simulink model "cosim_der2"  (R2021b)
settings: Solver=VariableStepAuto  StartTime=0.0  StopTime=inf  FixedStep=1e-3  RelTol=1e-3
values from neighbouring files (symbols this model uses):
  data_in = [0.785293830964 0.808251211481 0.30791492871 0.0344445946687 0.179843791508 0.360027135025 0.556566365757 0.556566365757 0.360027135025 0.179843791508 0.0344445946687 0.30791492871 ... (14 elements, 2x7)]    [caca.mat]    (also in cosim1.m = readmatrix("data_in1.csv"); cosim2.m = readmatrix("data_in2.csv"))
undefined symbols (not defined in the file or in its folder): xc7vx485tffg1157
libraries: hdlBasic x14, hdlSSR x1, vmcUtilities x1
settings Model: Creator=fabus  LastModifiedBy=fabus
settings DataIOCC: ExternalInput=data_in

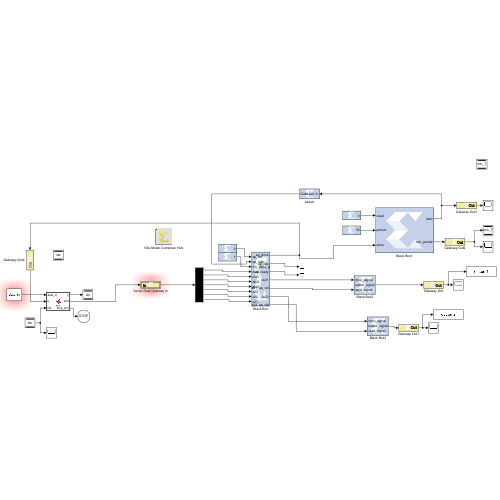
[thumbnail: Simulink's stored preview of the top-level diagram]
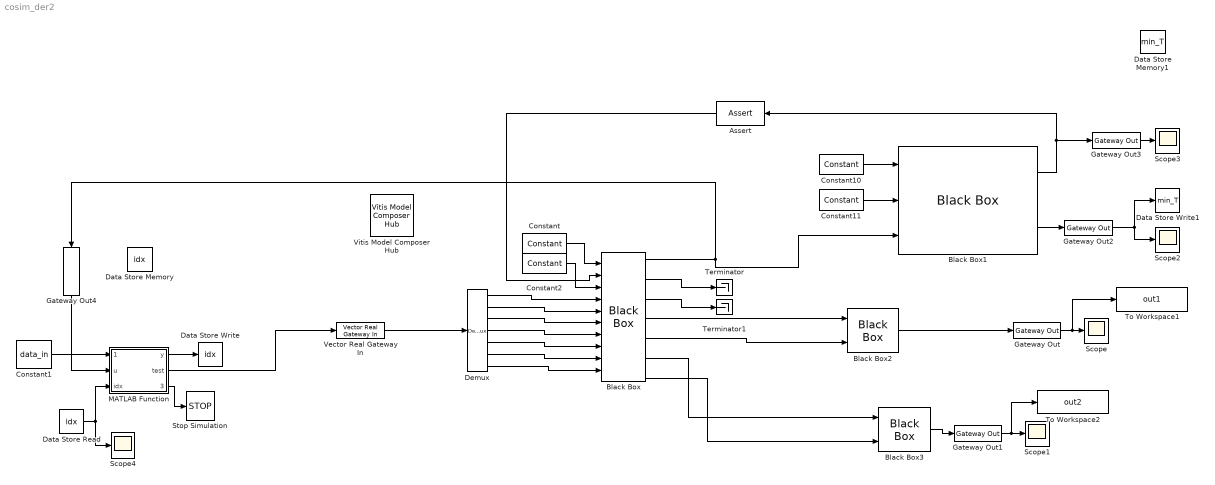
== system cosim_der2 ==
  Assert : hdlBasic/Assert  assert_type=off  type_source=Explicitly  gui_display_data_type=Fixed-point  arith_type=Signed (2's comp)  n_bits=16  bin_pt=14  preci_type=Single  exp_width=8  frac_width=24  assert_rate=on  rate_source=Explicitly  period=1  output_port=on  XmcBlockStatus=1  maskContainerNames=group1  block_type=assert  block_config=sysgen:assert_config  block_width=609  block_height=900
  Black Box : hdlBasic/Black Box  init_code=der2_config  sim_method=Vivado Simulator  verbose=off  XmcBlockStatus=1  maskContainerNames=group1  block_type=blackbox2  block_config=sysgen:black_box_config
  Black Box1 : hdlBasic/Black Box  init_code=period_setter_config  sim_method=Vivado Simulator  verbose=off  XmcBlockStatus=1  maskContainerNames=group1  block_type=blackbox2  block_config=sysgen:black_box_config
  Black Box2 : hdlBasic/Black Box  init_code=valid_out15_config  sim_method=Vivado Simulator  verbose=off  XmcBlockStatus=1  maskContainerNames=group1  block_type=blackbox2  block_config=sysgen:black_box_config
  Black Box3 : hdlBasic/Black Box  init_code=valid_out15_config  sim_method=Vivado Simulator  verbose=off  XmcBlockStatus=1  maskContainerNames=group1  block_type=blackbox2  block_config=sysgen:black_box_config
  Constant : hdlBasic/Constant  const=0  gui_display_data_type=Fixed-point  arith_type=Unsigned  n_bits=1  bin_pt=0  preci_type=Single  exp_width=8  frac_width=24  explicit_period=off  period=1  XmcBlockStatus=1  maskContainerNames=tabcontainer1  block_type=constant  block_config=sysgen:Constant_config
  Constant1 : Constant  Value=data_in
  Constant10 : hdlBasic/Constant  const=0  gui_display_data_type=Fixed-point  arith_type=Unsigned  n_bits=1  bin_pt=0  preci_type=Single  exp_width=8  frac_width=24  explicit_period=off  period=1  XmcBlockStatus=1  maskContainerNames=tabcontainer1  block_type=constant  block_config=sysgen:Constant_config
  Constant11 : hdlBasic/Constant  const=30  gui_display_data_type=Fixed-point  arith_type=Unsigned  n_bits=32  bin_pt=0  preci_type=Single  exp_width=8  frac_width=24  explicit_period=off  period=1  XmcBlockStatus=1  maskContainerNames=tabcontainer1  block_type=constant  block_config=sysgen:Constant_config
  Constant2 : hdlBasic/Constant  const=1  gui_display_data_type=Fixed-point  arith_type=Unsigned  n_bits=1  bin_pt=0  preci_type=Single  exp_width=8  frac_width=24  explicit_period=off  period=1  XmcBlockStatus=1  maskContainerNames=tabcontainer1  block_type=constant  block_config=sysgen:Constant_config
  Data Store Memory : DataStoreMemory  DataStoreName=idx  ReadBeforeWriteMsg=warning  WriteAfterWriteMsg=warning  WriteAfterReadMsg=warning  InitialValue=1  ShowAdditionalParam=off
  Data Store Memory1 : DataStoreMemory  DataStoreName=min_T  ReadBeforeWriteMsg=warning  WriteAfterWriteMsg=warning  WriteAfterReadMsg=warning  ShowAdditionalParam=off
  Data Store Read : DataStoreRead  DataStoreName=idx  IndexOptions=Index vector (dialog)  Indices=1  OutputSizes=1
  Data Store Write : DataStoreWrite  DataStoreName=idx  IndexOptions=Index vector (dialog)  Indices=1  OutputSizes=1
  Data Store Write1 : DataStoreWrite  DataStoreName=min_T  IndexOptions=Index vector (dialog)  Indices=1  OutputSizes=1
  Demux : Demux  Outputs=7
  Gateway Out{,1..3} (4 alike) : hdlBasic/Gateway Out  inherit_from_input=on  hdl_port=on  rows=1  columns=1  UseAsDAC=off  DACChannel='1'  interface=None  automatic_assignment=on  address_offset=hex2dec('00')  intf_name=''  intf_description=''  timing_constraint=None  locs_specified=off  LOCs={}  io_standard={}  XmcBlockStatus=1  maskContainerNames=group4  block_type=gatewayout  block_config=sysgen:gateway_out_config  block_width_w=590  block_height_w=620  block_width=620  block_height=750
  Gateway Out4 : hdlBasic/Gateway Out  inherit_from_input=off  hdl_port=off  rows=1  columns=1  UseAsDAC=off  DACChannel='1'  interface=None  automatic_assignment=on  address_offset=hex2dec('00')  intf_name=''  intf_description=''  timing_constraint=None  locs_specified=off  LOCs={}  io_standard={}  XmcBlockStatus=1  maskContainerNames=group4  block_type=gatewayout  block_config=sysgen:gateway_out_config  block_width_w=590  block_height_w=620  block_width=620  block_height=750
  MATLAB Function : MATLAB Function  TreatAsAtomicUnit=on
  Scope{,1..4} (5 alike) : Scope
  Stop Simulation : Stop
  Terminator : Terminator
  Terminator1 : Terminator
  To Workspace1 : ToWorkspace  VariableName=out1  SampleTime=31
      settings: Save2DSignal=2-D array (concatenate along first dimension)
  To Workspace2 : ToWorkspace  VariableName=out2  SampleTime=31
      settings: Save2DSignal=2-D array (concatenate along first dimension)
  Vector Real Gateway In : hdlSSR/Vector Real Gateway In  gui_display_data_type=Fixed-point  arith_type=Signed (2's comp)  n_bits=W  bin_pt=fr_width  preci_type=Single  exp_width=8  frac_width=24  quantization="Round  (unbiased: +/- Inf)"  overflow=Saturate  period=1  sg_ssr=7  UseAsADC=off  ADCChannel='1'  interface=None  automatic_assignment=on  address_offset=hex2dec('00')  intf_name=''  intf_description=''  default_value=0  timing_constraint=None  locs_specified=off  LOCs={}  io_standard={}  inherit_from_input=off  hdl_port=on  interface_prev=1  block_type=realgatewayin_ssr  XmcBlockStatus=1  sg_ssr_prev=7  maskContainerNames=group4  block_width_w=590  block_height_w=670  block_width=640  block_height=850
  Vitis Model Composer Hub : vmcUtilities/Vitis Model Composer Hub  Tag=genX  CodeGeneration=off  TargetDirectory=./code  ExportType=AI Engines  IpVendor=xilinx.com  IpLibrary=hls  IpVersion=1.0  IpHWLanguage=Verilog  AieCompilerOptions={}  CreateTestbench=off  TestbenchStackSize=10  RunAieSim=off  AieSimTimeout=50000  RunAieSimProfiling=off  LaunchVitisAnalyzer=off  PlotOutput=off  RunX86Sim=off  X86SimTimeout=10  GenHwImage=off  PlatformType=Not Specified  HwSystemType=Baremetal  HwValidationTarget=hw  ProjDevice=xc7vx485tffg1157-3  ProjDevicePart=xc7vx485tffg1157-3  SamplePeriod=-1  ClockFrequency=200  DataPathParallelism=1  xilinxfamily=virtex7  part=xc7vx485t  speed=-3  package=ffg1157  directory=./netlist  testbench=off  incr_netlist=off  synthesis_tool=Vivado  clock_wrapper=Clock Enables  dbl_ovrd=According to Block Masks  dcm_input_clock_period=10  sysclk_period=10  simulink_period=1  eval_field=0
  wires:
  Constant/1 -> Black Box/1
  Black Box1/1 -> Gateway Out3/1, Assert/1
  Constant10/1 -> Black Box1/1
  Constant11/1 -> Black Box1/2
  Black Box/1 -> Black Box1/3, Gateway Out4/1
  Gateway Out2/1 -> Scope2/1, Data Store Write1/1
  Black Box1/2 -> Gateway Out2/1
  Gateway Out/1 -> To Workspace1/1, Scope/1
  Black Box2/1 -> Gateway Out/1
  Black Box/4 -> Black Box2/1
  Black Box/5 -> Black Box2/2
  Black Box3/1 -> Gateway Out1/1
  Gateway Out1/1 -> To Workspace2/1, Scope1/1
  Black Box/6 -> Black Box3/1
  Black Box/7 -> Black Box3/2
  Assert/1 -> Black Box/2
  Gateway Out3/1 -> Scope3/1
  MATLAB Function/1(y) -> Data Store Write/1
  Data Store Read/1 -> MATLAB Function/3(idx), Scope4/1
  Gateway Out4/1 -> MATLAB Function/2(u)
  MATLAB Function/2(test) -> Vector Real Gateway In/1
  Constant1/1 -> MATLAB Function/1(data_in)
  Vector Real Gateway In/1 -> Demux/1
  Demux/1 -> Black Box/4
  Demux/7 -> Black Box/10
  Demux/6 -> Black Box/9
  Demux/5 -> Black Box/8
  Demux/4 -> Black Box/7
  Demux/3 -> Black Box/6
  Demux/2 -> Black Box/5
  Black Box/2 -> Terminator/1
  Black Box/3 -> Terminator1/1
  MATLAB Function/3(stop_sim) -> Stop Simulation/1
  Constant2/1 -> Black Box/3

== matlab function cosim_der2/MATLAB Function ==
  data: data_in input; u input; y output size=1; idx input; test output; stop_sim output
function [y, test, stop_sim] = fcn(data_in, u, idx)

%Detener simulación
stop_sim = 0;
persistent ndata
if isempty(ndata)
    ndata = length(data_in);
end
if(idx == ndata+2)
    disp('100%');
    fprintf('%d datos procesados exitosamente\n',int64(ndata));
    stop_sim = 1;
end

%Progreso
persistent avisar_sig
if isempty(avisar_sig)
    avisar_sig = 0.01;
end
if(idx/ndata > avisar_sig)
    fprintf('%3.0f %%\n', (avisar_sig*100));
    avisar_sig = avisar_sig + 0.01;
    if(avisar_sig > 1)
        avisar_sig = idx;
    end
end

%Sacar datos
y=idx;
if(u==1)
    y = idx+1;
end
test = flip(data_in(min(idx,ndata),:));
